simulink model "Direct_Realization_of_FIR_Fi"  (R2020a)
settings: Solver=VariableStepAuto  StartTime=0.0  StopTime=10.0  RelTol=1e-3
settings Model: Creator=tanu  LastModifiedBy=tanu
settings DataIOCC: SaveOutput=off  SaveTime=off

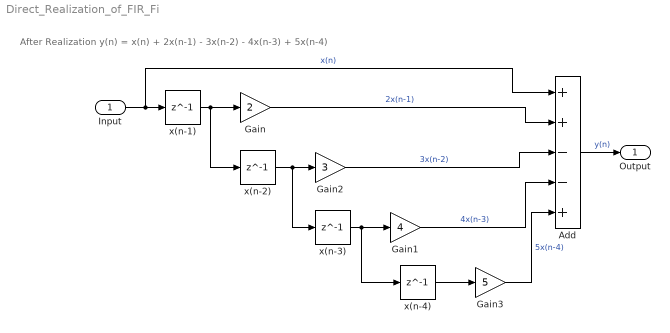
== system Direct_Realization_of_FIR_Fi ==
  note: After Realization y(n) = x(n) + 2x(n-1) - 3x(n-2) - 4x(n-3) + 5x(n-4)
  Input : Inport
  Add : Sum  Inputs=++--+
  Gain : Gain  Gain=2
  Gain1 : Gain  Gain=4
  Gain2 : Gain  Gain=3
  Gain3 : Gain  Gain=5
  x(n-1) : Delay  DelayLength=1
  x(n-2) : Delay  DelayLength=1
  x(n-3) : Delay  DelayLength=1
  x(n-4) : Delay  DelayLength=1
  Output : Outport
  wires:
  Input/1 -> Add/1, x(n-1)/1  "x(n)"
  x(n-3)/1 -> x(n-4)/1, Gain1/1
  x(n-4)/1 -> Gain3/1
  Gain3/1 -> Add/5  "5x(n-4)"
  x(n-1)/1 -> x(n-2)/1, Gain/1
  Gain2/1 -> Add/3  "3x(n-2)"
  Add/1 -> Output/1  "y(n)"
  x(n-2)/1 -> x(n-3)/1, Gain2/1
  Gain1/1 -> Add/4  "4x(n-3)"
  Gain/1 -> Add/2  "2x(n-1)"
